simulink model "stage1_motor_plant"  (R2026a)
settings: Solver=ode45  StopTime=0.5
undefined symbols (not defined in the file): B, J, Ke, Kt, L, R, TL
settings Model: Creator=knavn  LastModifiedBy=knavn

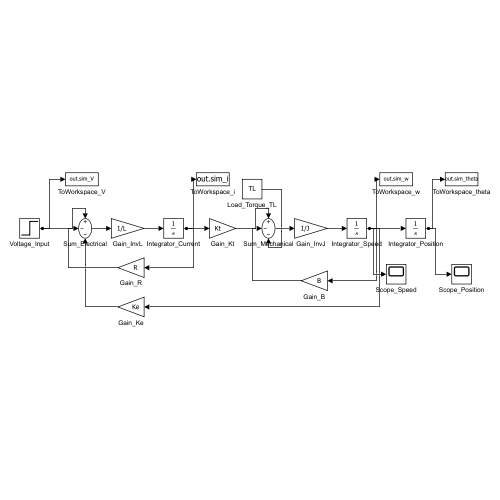
[thumbnail: Simulink's stored preview of the top-level diagram]
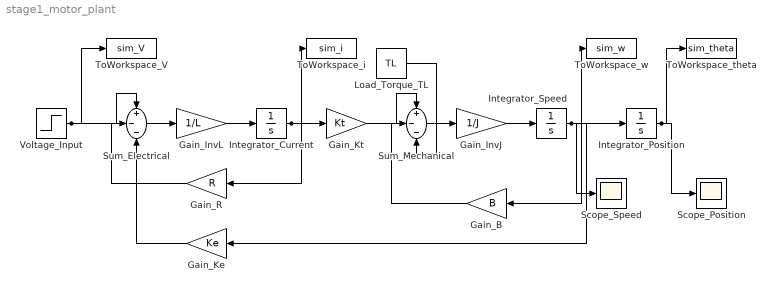
== system stage1_motor_plant ==
  Gain_B : Gain  Gain=B
  Gain_InvJ : Gain  Gain=1/J
  Gain_InvL : Gain  Gain=1/L
  Gain_Ke : Gain  Gain=Ke
  Gain_Kt : Gain  Gain=Kt
  Gain_R : Gain  Gain=R
  Integrator_Current : Integrator
  Integrator_Position : Integrator
  Integrator_Speed : Integrator
  Load_Torque_TL : Constant  Value=TL
  Scope_Position : Scope
  Scope_Speed : Scope
  Sum_Electrical : Sum  Inputs=+--
  Sum_Mechanical : Sum  Inputs=+--
  ToWorkspace_V : ToWorkspace  VariableName=sim_V  SaveFormat=Timeseries  SampleTime=-1
  ToWorkspace_i : ToWorkspace  VariableName=sim_i  SaveFormat=Timeseries  SampleTime=-1
  ToWorkspace_theta : ToWorkspace  VariableName=sim_theta  SaveFormat=Timeseries  SampleTime=-1
  ToWorkspace_w : ToWorkspace  VariableName=sim_w  SaveFormat=Timeseries  SampleTime=-1
  Voltage_Input : Step  Time=0.05  FinalValue=12  SampleTime=0
  wires:
  Voltage_Input/1 -> Sum_Electrical/1, ToWorkspace_V/1
  Sum_Electrical/1 -> Gain_InvL/1
  Gain_InvL/1 -> Integrator_Current/1
  Integrator_Current/1 -> Gain_R/1, Gain_Kt/1, ToWorkspace_i/1
  Gain_R/1 -> Sum_Electrical/2
  Gain_Kt/1 -> Sum_Mechanical/1
  Load_Torque_TL/1 -> Sum_Mechanical/3
  Sum_Mechanical/1 -> Gain_InvJ/1
  Gain_InvJ/1 -> Integrator_Speed/1
  Integrator_Speed/1 -> Gain_B/1, Gain_Ke/1, Integrator_Position/1, ToWorkspace_w/1, Scope_Speed/1
  Gain_B/1 -> Sum_Mechanical/2
  Gain_Ke/1 -> Sum_Electrical/3
  Integrator_Position/1 -> ToWorkspace_theta/1, Scope_Position/1
